simulink subsystem "iter_modulator"  (R2022a)
settings: Solver=VariableStepAuto  StartTime=0.0  StopTime=10.0  RelTol=1e-3
values from neighbouring files (symbols this model uses):
  dataNum = 16    [initSefdmModel.m]
  indiciesWithCP = [issuedSize-cpLength+1:issuedSize, 1:issuedSize]    [initSefdmModel.m]
  paddingN1 = fftSize - (N1+2)    (= 256)    [initSefdmModel.m]
libraries: dspxfrm3 x1, dspindex x1
settings Model: Creator=lsfan  LastModifiedBy=lsfan

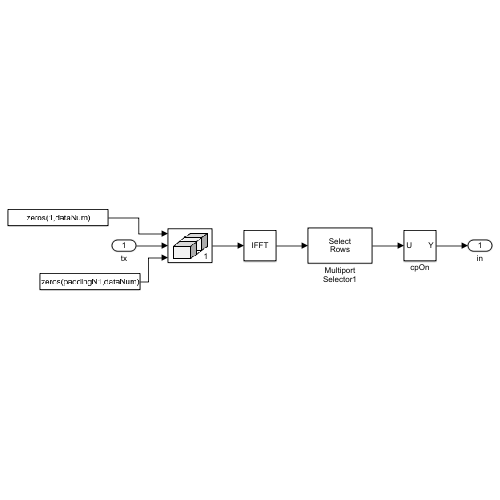
[thumbnail: Simulink's stored preview of the top-level diagram]
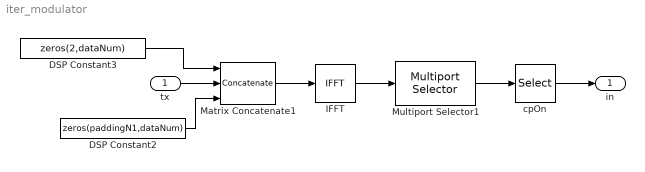
== system iter_modulator ==
  tx : Inport
  DSP Constant2 : Constant  Value=zeros(paddingN1,dataNum)  VectorParams1D=off  FramePeriod=Inf
      settings: SamplingMode=Frame based
  DSP Constant3 : Constant  Value=zeros(2,dataNum)  VectorParams1D=off  FramePeriod=Inf
      settings: SamplingMode=Frame based
  IFFT : dspxfrm3/IFFT  FFTImplementation=Auto  CompMethod=Table lookup  TableOpt=NEW  TableOptActive=Speed  BitRevOrder=off  cs_in=on  Normalize=on  InheritFFTLength=on  FFTLength=64  WrapInput=on  mode=Complex  outSamplingMode=Sample based  roundingMode=Floor  overflowMode=off  firstCoeffDataTypeStr=Inherit: Same word length as input  firstCoeffLastDataTypeStr=Inherit: Same word length as input  outputMin=[]  outputMax=[]
  Matrix Concatenate1 : Concatenate  NumInputs=3  Mode=Multidimensional array
  Multiport Selector1 : dspindex/Multiport Selector  rowsOrCols=Rows  idxCellArray={channelIssued}  idxErrMode=Clip Index
  cpOn : Selector  NumberOfDimensions=2  InputPortWidth=3  IndexOptions=Index vector (dialog),Select all  Indices=indiciesWithCP,indiciesWithCP  OutputSizes=1,1
  in : Outport
  wires:
  DSP Constant2/1 -> Matrix Concatenate1/3
  DSP Constant3/1 -> Matrix Concatenate1/1
  tx/1 -> Matrix Concatenate1/2
  cpOn/1 -> in/1
  Multiport Selector1/1 -> cpOn/1
  IFFT/1 -> Multiport Selector1/1
  Matrix Concatenate1/1 -> IFFT/1
